simulink model "Modello_SIM"  (R2015a)
settings: Solver=ode45  StartTime=0.0  StopTime=10.0  RelTol=1e-3
settings Model: Creator=edo  LastModifiedBy=edo

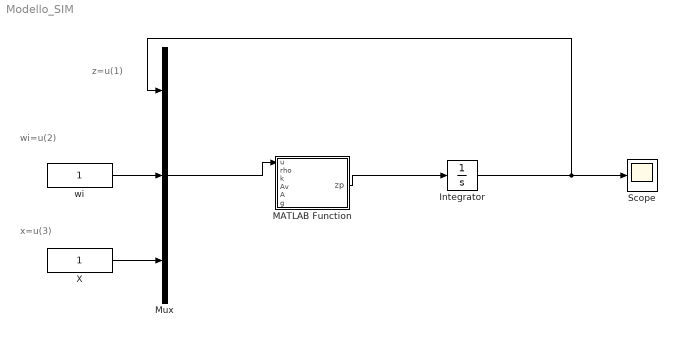
== system Modello_SIM ==
  note: x=u(3)
  note: wi=u(2)
  note: z=u(1)
  Integrator : Integrator
  MATLAB Function : MATLAB Function  TreatAsAtomicUnit=on
  Mux : Mux  Inputs=3
  Scope : Scope
  "X " : FromWorkspace  VariableName=1  SampleTime=0
  "wi " : FromWorkspace  VariableName=1  SampleTime=0
  wires:
  Mux/1 -> MATLAB Function/1(u)
  MATLAB Function/1(zp) -> Integrator/1
  Integrator/1 -> Mux/1, Scope/1
  "wi "/1 -> Mux/2
  "X "/1 -> Mux/3

== matlab function Modello_SIM/MATLAB Function ==
  data: u input; zp output; rho input; k input; Av input; A input; g input
% function that return the derivative of the liquid livel in the tank
function zp  = model(u,rho,k,Av,A,g)
z = u(1);
model.m
% first input: tank level
wi = u(2); % second input: input flow rate
x = min(1,max(0,u(3))); % third input: stem position 0<=x<=1
zp = (wi/(rho*A))-k*(Av/A)*x*sqrt(g)*sqrt(z); %  z_point expression
